simulink model "legBE"  (Simulink 8.8)
settings: Solver=VariableStepAuto  StartTime=0.0  StopTime=10.0  RelTol=1e-3
settings Model: Creator=Ctamp  LastModifiedBy=Ctamp
settings DataIOCC: LimitDataPoints=off  SaveFormat=Dataset  SignalLoggingSaveFormat=Dataset
settings OptimizationCC: LifeSpan=auto
settings DebuggingCC: UnderspecifiedInitializationDetection=Simplified  MergeDetectMultiDrivingBlocksExec=error  FcnCallInpInsideContextMsg=error  StateNameClashWarn=none  SFUnexpectedBacktrackingDiag=error  SFNoUnconditionalDefaultTransitionDiag=error  SFExecutionAtInitializationDiag=warning
settings HardwareCC: ProdBitPerPointer=64  ProdBitPerSizeT=64  ProdBitPerPtrDiffT=64  ProdLargestAtomicFloat=Float  ProdIntDivRoundTo=Zero  ProdEndianess=LittleEndian  ProdWordSize=64  ProdHWDeviceType=Intel->x86-64 (Windows64)
settings ModelReferenceCC: PropagateSignalLabelsOutOfModel=on
settings GRTTargetCC: TargetLangStandard=C99 (ISO)  GeneratePreprocessorConditionals=Use local settings  CombineOutputUpdateFcns=on  GRTInterface=off
settings ConfigComp: CovMetricSettings=dwe  CovHtmlReporting=off  CovSaveCumulativeToWorkspaceVar=off  CovSaveSingleToWorkspaceVar=off  CovExternalEMLEnable=on

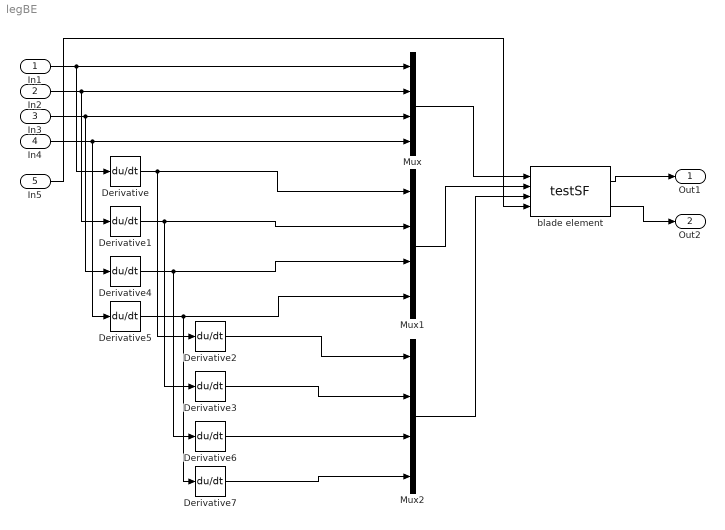
== system legBE ==
  In1 : Inport
  In2 : Inport  Port=2
  In3 : Inport  Port=3
  In4 : Inport  Port=4
  In5 : Inport  Port=5
  Derivative{,1..7} (8 alike) : Derivative
  Mux : Mux
  Mux1 : Mux
  Mux2 : Mux
  blade element : M-S-Function  FunctionName=testSF  Parameters=1
      mask Display: disp('blade element')
  Out1 : Outport
  Out2 : Outport  Port=2
  wires:
  blade element/1 -> Out1/1
  Mux/1 -> blade element/1
  Mux1/1 -> blade element/2
  Mux2/1 -> blade element/3
  In1/1 -> Derivative/1, Mux/1
  In2/1 -> Derivative1/1, Mux/2
  In3/1 -> Derivative4/1, Mux/3
  In4/1 -> Derivative5/1, Mux/4
  Derivative/1 -> Derivative2/1, Mux1/1
  Derivative1/1 -> Derivative3/1, Mux1/2
  Derivative4/1 -> Derivative6/1, Mux1/3
  Derivative5/1 -> Derivative7/1, Mux1/4
  Derivative2/1 -> Mux2/1
  Derivative3/1 -> Mux2/2
  Derivative6/1 -> Mux2/3
  Derivative7/1 -> Mux2/4
  In5/1 -> blade element/4
  blade element/2 -> Out2/1
